simulink model "Ex_7"  (Simulink 8.0)
settings: Solver=ode45  StartTime=0.0  StopTime=10.0  RelTol=1e-3
settings Model: Creator=Faradars  LastModifiedBy=Faradars

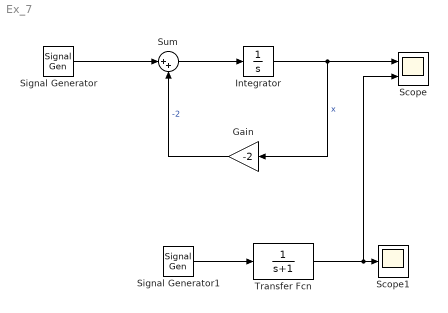
== system Ex_7 ==
  Gain : Gain  Gain=-2
  Integrator : Integrator
  Scope : Scope  NumInputPorts=2
      settings: YMin=-5~-5  YMax=5~5
  Scope1 : Scope
  Signal Generator : SignalGenerator  WaveForm=square
  Signal Generator1 : SignalGenerator  WaveForm=square
  Sum : Sum  Inputs=|++
  Transfer Fcn : TransferFcn  Denominator=[1 1]
  wires:
  Signal Generator/1 -> Sum/1
  Sum/1 -> Integrator/1
  Integrator/1 -> Scope/1, Gain/1  "x"
  Gain/1 -> Sum/2  "-2"
  Signal Generator1/1 -> Transfer Fcn/1
  Transfer Fcn/1 -> Scope/2, Scope1/1
